simulink model "Practia1si"  (R2025a)
settings: Solver=VariableStepAuto  StartTime=0.0  StopTime=10.0  RelTol=1e-3

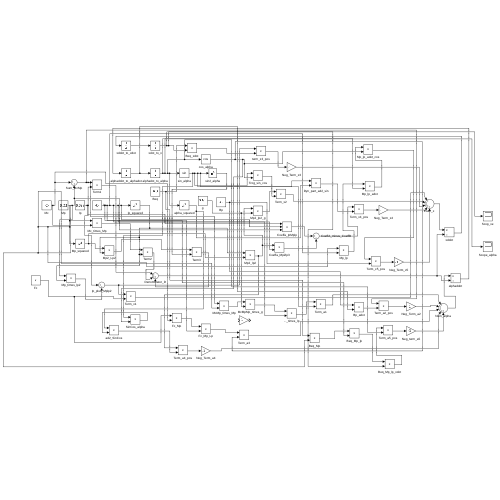
[thumbnail: Simulink's stored preview of the top-level diagram]
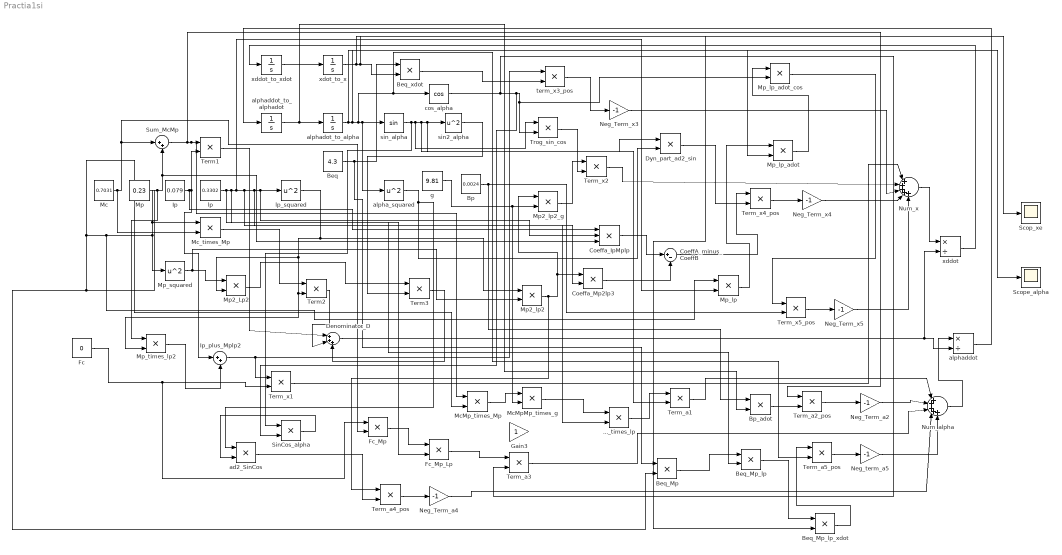
== system Practia1si ==
  ..._times_lp : Product
  Beq : Constant  Value=4.3
  Beq_Mp : Product
  Beq_Mp_lp : Product
  Beq_Mp_lp_xdot : Product
  Beq_xdot : Product
  Bp : Constant  Value=0.0024
  Bp_adot : Product
  CoeffA_minus_CoeffB : Sum  Inputs=|+-
  Coeffa_IpMplp : Product  Inputs=3
  Coeffa_Mp2lp3 : Product
  Denominator_D : Sum  Inputs=|+++
  Dyn_part_ad2_sin : Product
  Fc : Constant  Value=0
  Fc_Mp : Product
  Fc_Mp_Lp : Product
  Gain3 : Gain
  Ip : Constant  Value=0.079
  Ip_plus_Mplp2 : Sum  Inputs=|++
  Mc : Constant  Value=0.7031
  McMpMp_times_g : Product
  McMp_times_Mp : Product
  Mc_times_Mp : Product
  Mp : Constant  Value=0.23
  Mp2_Lp2 : Product
  Mp2_lp2 : Product
  Mp2_lp2_g : Product
  Mp_lp : Product
  Mp_lp_adot : Product
  Mp_lp_adot_cos : Product
  Mp_squared : Math  Operator=square
  Mp_times_lp2 : Product
  Neg_Term_a2 : Gain  Gain=-1
  Neg_Term_a4 : Gain  Gain=-1
  Neg_Term_x3 : Gain  Gain=-1
  Neg_Term_x4 : Gain  Gain=-1
  Neg_Term_x5 : Gain  Gain=-1
  Neg_term_a5 : Gain  Gain=-1
  Num_alpha : Sum  Inputs=|+++++
  Num_x : Sum  Inputs=|+++++
  Scop_xe : Scope
      settings: ActiveDisplayYMinimum=-2.0957040519639394  ActiveDisplayYMaximum=11.180072654286743
  Scope_alpha : Scope
      settings: ActiveDisplayYMinimum=-96.260001472253833  ActiveDisplayYMaximum=78.042537029961892
  SinCos_alpha : Product
  Sum_McMp : Sum  Inputs=|++
  Term1 : Product
  Term2 : Product
  Term3 : Product
  Term_a1 : Product
  Term_a2_pos : Product
  Term_a3 : Product
  Term_a4_pos : Product
  Term_a5_pos : Product
  Term_x1 : Product
  Term_x2 : Product
  Term_x4_pos : Product
  Term_x5_pos : Product
  Trog_sin_cos : Product
  ad2_SinCos : Product
  alpha_squared : Math  Operator=square
  alphaddot : Product  Inputs=*/
  alphaddot_to_alphadot : Integrator  InitialCondition=pi/180
  alphadot_to_alpha : Integrator
  cos_alpha : Trigonometry  Operator=cos
  g : Constant  Value=9.81
  lp : Constant  Value=0.3302
  lp_squared : Math  Operator=square
  sin2_alpha : Math  Operator=square
  sin_alpha : Trigonometry
  term_x3_pos : Product
  xddot : Product  Inputs=*/
  xddot_to_xdot : Integrator
  xdot_to_x : Integrator
  wires:
  xddot_to_xdot/1 -> xdot_to_x/1
  alphaddot_to_alphadot/1 -> Bp_adot/2, alphadot_to_alpha/1
  lp/1 -> Beq_Mp_lp/2, Fc_Mp_Lp/2, Mp_lp/2, ..._times_lp/2, Coeffa_Mp2lp3/2, lp_squared/1, Coeffa_IpMplp/2
  Mc_times_Mp/1 -> Term2/1
  lp_squared/1 -> Term2/2, Mp_times_lp2/2, Mp2_Lp2/2, Mp2_lp2/1
  Mp_squared/1 -> Mp2_lp2/2, Mp2_Lp2/1
  alphadot_to_alpha/1 -> Mp_lp_adot/2, Scope_alpha/1, alpha_squared/1, sin_alpha/1, Term_a5_pos/2, cos_alpha/1
  Mp2_Lp2/1 -> Term3/1
  sin2_alpha/1 -> Term3/2
  Term1/1 -> Denominator_D/1
  Term2/1 -> Denominator_D/2
  Term3/1 -> Denominator_D/3
  Ip/1 -> Coeffa_IpMplp/1, Ip_plus_Mplp2/1, Term1/2
  Mp_times_lp2/1 -> Ip_plus_Mplp2/2
  Fc/1 -> Fc_Mp/1, Term_x1/2
  sin_alpha/1 -> SinCos_alpha/1, Trog_sin_cos/1, Term_a1/2, Dyn_part_ad2_sin/1, sin2_alpha/1
  cos_alpha/1 -> Term_a3/2, SinCos_alpha/2, Trog_sin_cos/2, Mp_lp_adot_cos/2
  Mp2_lp2/1 -> Term_a4_pos/1, Coeffa_Mp2lp3/1, Mp2_lp2_g/1
  g/1 -> McMpMp_times_g/2, Mp2_lp2_g/2
  Mp2_lp2_g/1 -> Term_x2/1
  Trog_sin_cos/1 -> Term_x2/2
  xdot_to_x/1 -> Scop_xe/1, Beq_Mp_lp_xdot/2, Beq_xdot/2
  Beq/1 -> Beq_Mp/1, Beq_xdot/1
  Beq_xdot/1 -> term_x3_pos/2
  Ip_plus_Mplp2/1 -> term_x3_pos/1, Term_x1/1
  term_x3_pos/1 -> Neg_Term_x3/1
  Mp/1 -> Beq_Mp/2, McMp_times_Mp/2, Mp_times_lp2/1, Coeffa_IpMplp/3, Sum_McMp/2, Mc_times_Mp/1, Mp_squared/1, Mp_lp/1
  Coeffa_IpMplp/1 -> CoeffA_minus_CoeffB/1
  Coeffa_Mp2lp3/1 -> CoeffA_minus_CoeffB/2
  alpha_squared/1 -> ad2_SinCos/1, Dyn_part_ad2_sin/2
  CoeffA_minus_CoeffB/1 -> Term_x4_pos/1
  Dyn_part_ad2_sin/1 -> Term_x4_pos/2
  Term_x4_pos/1 -> Neg_Term_x4/1
  Mp_lp/1 -> Mp_lp_adot/1
  Mp_lp_adot/1 -> Mp_lp_adot_cos/1
  Mp_lp_adot_cos/1 -> Term_x5_pos/1
  Bp/1 -> Bp_adot/1, Term_x5_pos/2
  Term_x5_pos/1 -> Neg_Term_x5/1
  Term_x1/1 -> Num_x/1
  Term_x2/1 -> Num_x/2
  Neg_Term_x3/1 -> Num_x/3
  Neg_Term_x4/1 -> Num_x/4
  Neg_Term_x5/1 -> Num_x/5
  Num_x/1 -> xddot/1
  Denominator_D/1 -> alphaddot/2, xddot/2
  xddot/1 -> xddot_to_xdot/1
  McMp_times_Mp/1 -> McMpMp_times_g/1
  McMpMp_times_g/1 -> ..._times_lp/1
  ..._times_lp/1 -> Term_a1/1
  Bp_adot/1 -> Term_a2_pos/2
  Sum_McMp/1 -> Term_a2_pos/1, McMp_times_Mp/1, Term1/1
  Term_a2_pos/1 -> Neg_Term_a2/1
  Mc/1 -> Mc_times_Mp/2, Fc_Mp/2, Sum_McMp/1
  Fc_Mp/1 -> Fc_Mp_Lp/1
  Fc_Mp_Lp/1 -> Term_a3/1
  SinCos_alpha/1 -> ad2_SinCos/2
  ad2_SinCos/1 -> Term_a4_pos/2
  Term_a4_pos/1 -> Neg_Term_a4/1
  Beq_Mp/1 -> Beq_Mp_lp/1
  Beq_Mp_lp/1 -> Beq_Mp_lp_xdot/1
  Beq_Mp_lp_xdot/1 -> Term_a5_pos/1
  Term_a5_pos/1 -> Neg_term_a5/1
  Term_a1/1 -> Num_alpha/1
  Neg_Term_a2/1 -> Num_alpha/2
  Term_a3/1 -> Num_alpha/3
  Neg_Term_a4/1 -> Num_alpha/4
  Neg_term_a5/1 -> Num_alpha/5
  Num_alpha/1 -> alphaddot/1
  alphaddot/1 -> alphaddot_to_alphadot/1
